simulink model "MVEM"  (Simulink 8.1)
settings: Solver=ode15s  StartTime=0  StopTime=100  FixedStep=1e-3  RelTol=1e-5  AbsTol=1e-5
undefined symbols (not defined in the file or in its folder): generators
libraries: EngineSystemSubmodel x3, simulink x1, gensetMV x1
settings Model: Creator=yum  LastModifiedBy=yum
settings DataIOCC: SaveFormat=StructureWithTime  SignalLoggingSaveFormat=Dataset  InspectSignalLogs=on  ReturnWorkspaceOutputs=on
settings OptimizationCC: ExpressionDepthLimit=128
settings DebuggingCC: SolverPrmCheckMsg=none  FcnCallInpInsideContextMsg=EnableAllAsError
settings GRTTargetCC: CombineOutputUpdateFcns=on  GRTInterface=off

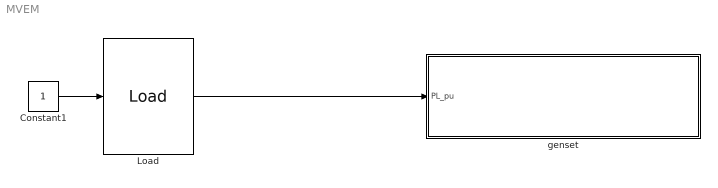
== system MVEM ==
  Constant1 : Constant
  Load : EngineSystemSubmodel/Load  Load_index=Load_index  Load_amp=Load_amp  Load_bias=Load_bias  Start_time=Start_time  T_load=T_load
  genset : Subsystem  mask{genset=generators(1)}
      mask prompts: genset "Generator parameters"
  wires:
  Load/1 -> genset/1(PL_pu)
  Constant1/1 -> Load/1

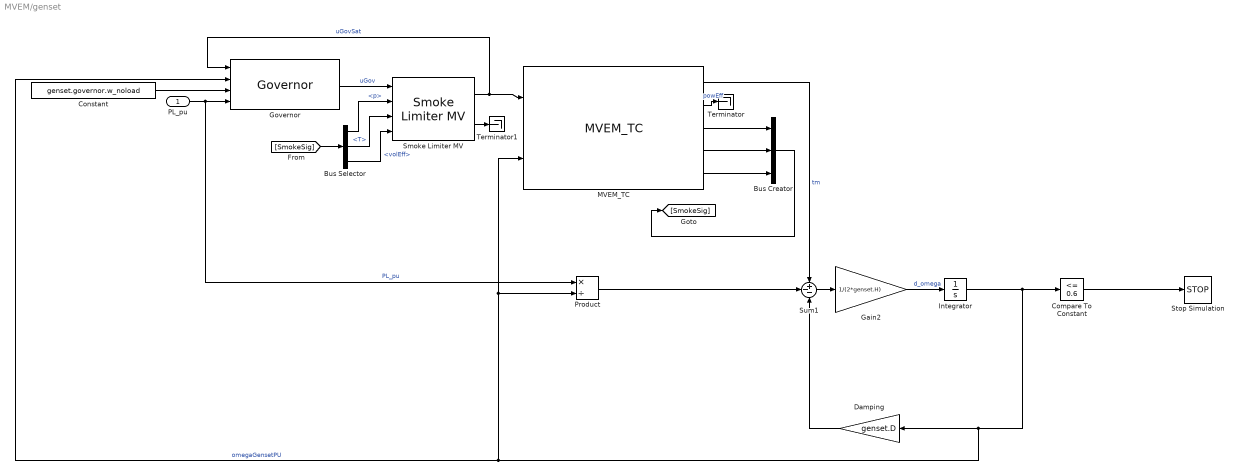
== system MVEM/genset ==
  PL_pu : Inport
  Bus Creator : BusCreator  Inputs=3
  Bus Selector : BusSelector  OutputSignals=p,T,volEff
  Compare To Constant : simulink/Logic and Bit Operations/Compare To Constant  relop=<=  const=0.6  OutDataTypeStr=boolean
  Constant : Constant  Value=genset.governor.w_noload
  Damping : Gain  Gain=genset.D
  Gain2 : Gain  Gain=1/(2*genset.H)
  Governor : gensetMV/GensetAC_MVM/Genset/Governor
  Integrator : Integrator  InitialCondition=generators(1).omega0
  MVEM_TC : EngineSystemSubmodel/MVEM_TC  genset=genset
  Product : Product  Inputs=*/
  Smoke Limiter MV : EngineSystemSubmodel/Smoke Limiter MV  fs=genset.eng.fs  Vd=genset.eng.vD  F_max=genset.eng.fMax  m_f_cyc_max=genset.eng.mFCycMax
  Stop Simulation : Stop
  Sum1 : Sum  Inputs=+--
  Terminator : Terminator
  Terminator1 : Terminator
  wires:
  Sum1/1 -> Gain2/1
  Gain2/1 -> Integrator/1  "d_omega"
  MVEM_TC/4 -> Bus Creator/2
  Governor/1 -> Smoke Limiter MV/1  "uGov"
  Integrator/1 -> Compare To Constant/1, Governor/2, MVEM_TC/2, Product/2, Damping/1  "omegaGensetPU"
  MVEM_TC/2 -> Terminator/1  "powEff"
  Smoke Limiter MV/2 -> Terminator1/1
  Constant/1 -> Governor/3
  MVEM_TC/1 -> Sum1/1  "tm"
  Damping/1 -> Sum1/3
  Bus Creator/1 -> [SmokeSig]
  Product/1 -> Sum1/2
  PL_pu/1 -> Product/1, Governor/4  "PL_pu"
  Smoke Limiter MV/1 -> MVEM_TC/1, Governor/1  "uGovSat"
  [SmokeSig] -> Bus Selector/1
  MVEM_TC/3 -> Bus Creator/1
  Compare To Constant/1 -> Stop Simulation/1
  MVEM_TC/5 -> Bus Creator/3
  Bus Selector/2 -> Smoke Limiter MV/3  "<T>"
  Bus Selector/1 -> Smoke Limiter MV/2  "<p>"
  Bus Selector/3 -> Smoke Limiter MV/4  "<volEff>"
